simulink model "gps_simulate_visibility_demo"  (Simulink 7.3)
settings: Solver=ode45  StartTime=0.0  StopTime=86400  RelTol=1e-3
undefined symbols (not defined in the file): WGS
libraries: rapidstm32_gps_lib x7
settings Model: Creator=Compaq  LastModifiedBy=Compaq

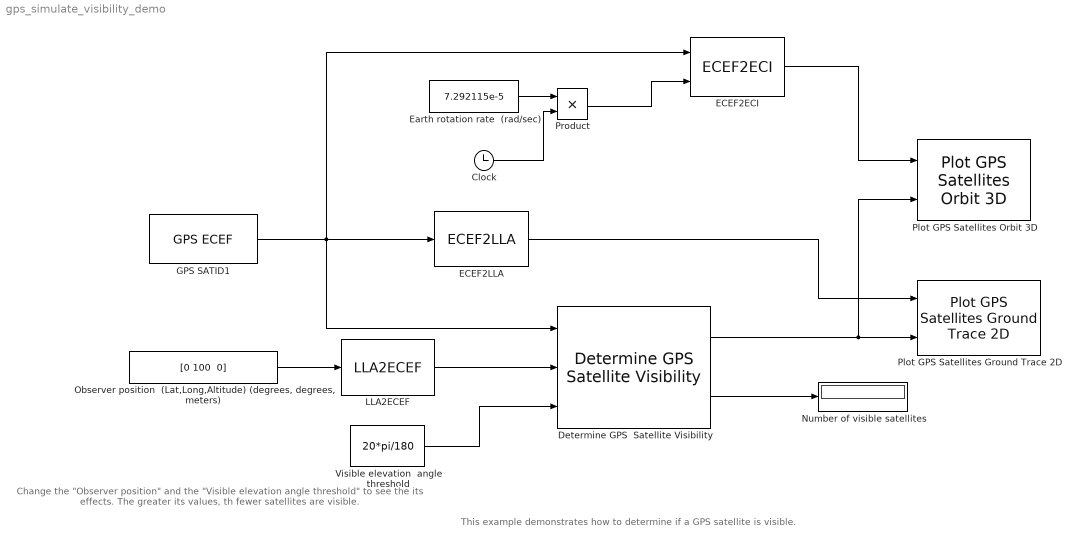
== system gps_simulate_visibility_demo ==
  note: This example demonstrates how to determine if a GPS satellite is visible.
  note: Change the "Observer position"
      | and the "Visible elevation
      | angle threshold"
      | to see the its effects.
      | The greater its values,
      | th fewer satellites are visible.
  Clock : Clock
      settings: Decimation=10
  Determine GPS  Satellite Visibility : rapidstm32_gps_lib/Determine GPS  Satellite Visibility
  ECEF2ECI : rapidstm32_gps_lib/ECEF2ECI
  ECEF2LLA : rapidstm32_gps_lib/ECEF2LLA  latlong_format=Degrees  altitude_format=Meters  refellipsoid=WGS-84  re=6378137  epsilon=0.081819190842622
  Earth rotation rate  (rad/sec) : Constant  Value=7.292115e-5  OutDataType=fixdt(1, 16)  OutScaling=2^0
  GPS SATID1 : rapidstm32_gps_lib/GPS ECEF  satid=All 24  t0=0  sampletime=600
  LLA2ECEF : rapidstm32_gps_lib/LLA2ECEF  latlong_format=Degrees  refellipsoid=WGS-84  re=6378137  epsilon=0.081819190842622
  Number of visible satellites : Display
  "Observer position  (Lat,Long,Altitude) (degrees, degrees, meters)" : Constant  Value="[0 100  0]"  OutDataType=fixdt(1, 16)  OutScaling=2^0
  Plot GPS Satellites Ground Trace 2D : rapidstm32_gps_lib/Plot GPS Satellites Ground Trace 2D  satid_all=on  satid1=on  satid2=on  satid3=on  satid4=on  satid5=on  satid6=on  satid7=on  satid8=on  satid9=on  satid10=on  satid11=on  satid12=on  satid13=on  satid14=on  satid15=on  satid16=on  satid17=on  satid18=on  satid19=on  satid20=on  satid21=on  satid22=on  satid23=on  satid24=on  visibility_vec=Yes
  Plot GPS Satellites Orbit 3D : rapidstm32_gps_lib/Plot GPS Satellites Orbit 3D  satid_all=on  satid1=on  satid2=on  satid3=on  satid4=on  satid5=on  satid6=on  satid7=on  satid8=on  satid9=on  satid10=on  satid11=on  satid12=on  satid13=on  satid14=on  satid15=on  satid16=on  satid17=on  satid18=on  satid19=on  satid20=on  satid21=on  satid22=on  satid23=on  satid24=on  visibility_vec=Yes
  Product : Product  OutDataType=fixdt(1, 16)  OutScaling=2^0  RndMeth=Zero
  Visible elevation  angle threshold : Constant  Value=20*pi/180  OutDataType=fixdt(1, 16)  OutScaling=2^0
  wires:
  GPS SATID1/1 -> ECEF2LLA/1, ECEF2ECI/1, Determine GPS  Satellite Visibility/1
  "Observer position  (Lat,Long,Altitude) (degrees, degrees, meters)"/1 -> LLA2ECEF/1
  LLA2ECEF/1 -> Determine GPS  Satellite Visibility/2
  Determine GPS  Satellite Visibility/1 -> Plot GPS Satellites Orbit 3D/2, Plot GPS Satellites Ground Trace 2D/2
  ECEF2LLA/1 -> Plot GPS Satellites Ground Trace 2D/1
  ECEF2ECI/1 -> Plot GPS Satellites Orbit 3D/1
  Earth rotation rate  (rad/sec)/1 -> Product/1
  Clock/1 -> Product/2
  Product/1 -> ECEF2ECI/2
  Determine GPS  Satellite Visibility/2 -> Number of visible satellites/1
  Visible elevation  angle threshold/1 -> Determine GPS  Satellite Visibility/3
